simulink model "LMS_FILTER_8_TAP"  (R2016a)
settings: Solver=VariableStepAuto  StartTime=0.0  StopTime=4000  RelTol=1e-3
libraries: dspsrcs4 x2, dspstat3 x2, dspmathops x1
settings Model: Creator=HP  LastModifiedBy=HP

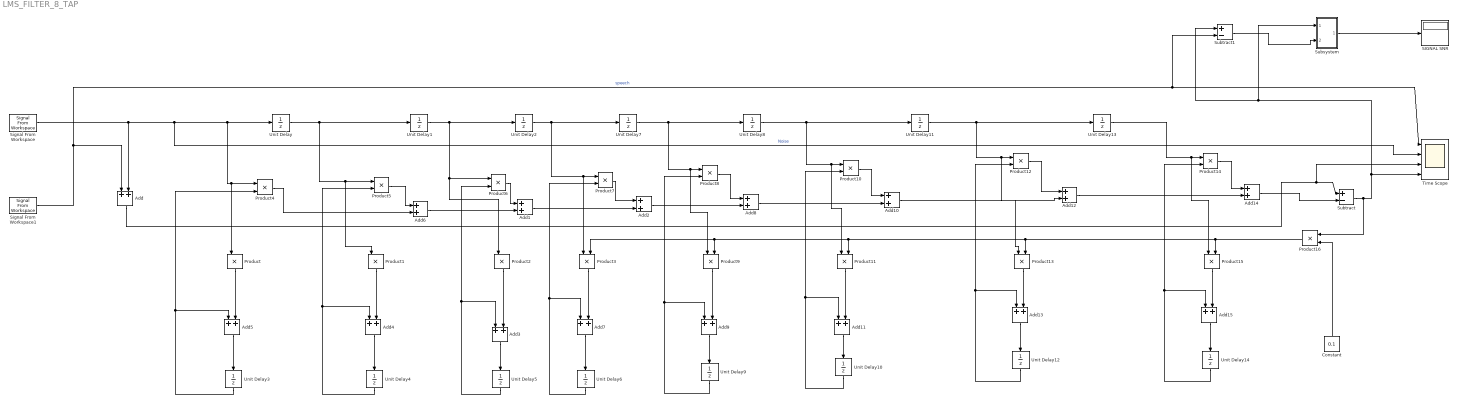
== system LMS_FILTER_8_TAP ==
  Add{,1..15} (16 alike) : Sum
  Constant : Constant  Value=0.1
  Product{,1..16} (17 alike) : Product
  "SIGNAL SNR " : Display
  Signal From Workspace : dspsrcs4/Signal From Workspace  X=n  Ts=1  nsamps=1  OutputAfterFinalValue=Setting to zero  ignoreOrWarnInputAndFrameLengths=off  OutputFrames=off
  Signal From Workspace1 : dspsrcs4/Signal From Workspace  X=s  Ts=1  nsamps=1  OutputAfterFinalValue=Setting to zero  ignoreOrWarnInputAndFrameLengths=off  OutputFrames=off
  Subsystem : Subsystem
  Subtract : Sum  Inputs=+-
  Subtract1 : Sum  Inputs=+-
  Time Scope : Scope  NumInputPorts=4
  Unit Delay{,1..14} (15 alike) : UnitDelay  SampleTime=-1
  wires:
  Unit Delay/1 -> Unit Delay1/1, Product5/1, Product1/1
  Unit Delay1/1 -> Product2/1, Product6/1, Unit Delay2/1
  Unit Delay2/1 -> Unit Delay7/1, Product7/1, Product3/1
  Unit Delay3/1 -> Add5/1, Product4/2
  Product/1 -> Add5/2
  Unit Delay4/1 -> Add4/1, Product5/2
  Add5/1 -> Unit Delay3/1
  Add4/1 -> Unit Delay4/1
  Product1/1 -> Add4/2
  Product5/1 -> Add6/1
  Product4/1 -> Add6/2
  Product2/1 -> Add3/2
  Unit Delay5/1 -> Add3/1, Product6/2
  Add3/1 -> Unit Delay5/1
  Product6/1 -> Add1/1
  Add6/1 -> Add1/2
  Unit Delay6/1 -> Add7/1, Product7/2
  Product3/1 -> Add7/2
  Product7/1 -> Add2/1
  Add1/1 -> Add2/2
  Add7/1 -> Unit Delay6/1
  Signal From Workspace/1 -> Add/2, Time Scope/2, Unit Delay/1, Product4/1, Product/1  "Noise"
  Unit Delay7/1 -> Unit Delay8/1, Product8/1, Product9/1
  Add9/1 -> Unit Delay9/1
  Unit Delay9/1 -> Add9/1, Product8/2
  Product8/1 -> Add8/1
  Add2/1 -> Add8/2
  Product9/1 -> Add9/2
  Unit Delay8/1 -> Unit Delay11/1, Product10/1, Product11/1
  Add11/1 -> Unit Delay10/1
  Unit Delay10/1 -> Add11/1, Product10/2
  Product10/1 -> Add10/1
  Add8/1 -> Add10/2
  Product11/1 -> Add11/2
  Unit Delay11/1 -> Unit Delay13/1, Product12/1, Product13/1
  Add13/1 -> Unit Delay12/1
  Unit Delay12/1 -> Add13/1, Product12/2
  Product12/1 -> Add12/1
  Add10/1 -> Add12/2
  Product13/1 -> Add13/2
  Unit Delay13/1 -> Product14/1, Product15/1
  Add15/1 -> Unit Delay14/1
  Unit Delay14/1 -> Add15/1, Product14/2
  Product14/1 -> Add14/1
  Add12/1 -> Add14/2
  Product15/1 -> Add15/2
  Add14/1 -> Subtract/2
  Add/1 -> Time Scope/3, Subtract/1
  Constant/1 -> Product16/2
  Product16/1 -> Product15/2, Product13/2, Product11/2, Product9/2, Product3/2
  Signal From Workspace1/1 -> Add/1, Time Scope/1, Subtract1/2  "speech"
  Subtract/1 -> Product16/1, Time Scope/4, Subsystem/1(In1), Subtract1/1
  Subtract1/1 -> Subsystem/2(In2)
  Subsystem/1(Out1) -> "SIGNAL SNR "/1

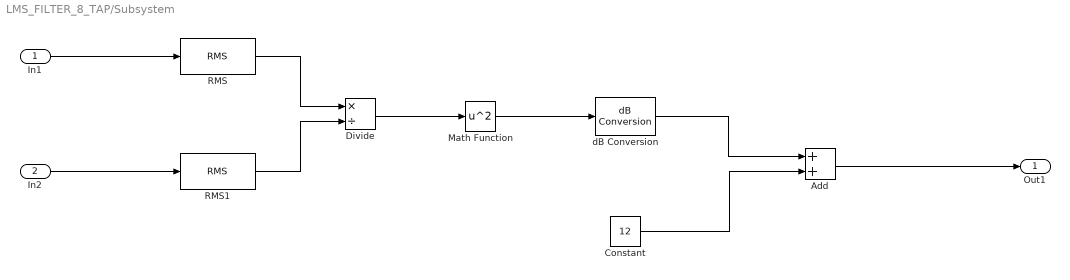
== system LMS_FILTER_8_TAP/Subsystem ==
  In1 : Inport
  In2 : Inport  Port=2
  Add : Sum
  Constant : Constant  Value=12
  Divide : Product  Inputs=*/
  Math Function : Math  Operator=square  OutputSignalType=real  SaturateOnIntegerOverflow=on
  RMS : dspstat3/RMS  run=on  reset_popup=None  InputProcessing=Columns as channels (frame based)  directionMode=Each column  dimension=1
  RMS1 : dspstat3/RMS  run=on  reset_popup=None  InputProcessing=Columns as channels (frame based)  directionMode=Each column  dimension=1
  dB Conversion : dspmathops/dB Conversion  dBtype=dB  intype=Amplitude  R=1  fuzz=off
  Out1 : Outport
  wires:
  RMS1/1 -> Divide/2
  dB Conversion/1 -> Add/1
  In1/1 -> RMS/1
  Divide/1 -> Math Function/1
  RMS/1 -> Divide/1
  In2/1 -> RMS1/1
  Add/1 -> Out1/1
  Constant/1 -> Add/2
  Math Function/1 -> dB Conversion/1
